simulink model "RegulationSim_v6_N8_5_States"  (R2019b)
settings: Solver=FixedStepAuto  StartTime=0.0  StopTime=100  FixedStep=0.1  RelTol=1e-3
values from neighbouring files (symbols this model uses):
  A = c.A    [MPC_u.m]    (also in base_lab4.m; mpc_regulation.m)
  B = c.B    [MPC_u.m]    (also in base_lab4.m; mpc_regulation.m)
  C = c.C    [MPC_u.m]    (also in base_lab4.m; mpc_regulation.m)
  D = 0    [MPC_u.m]    (also in base_lab4.m; mpc_regulation.m)
undefined symbols (not defined in the file or in its folder): A_new, B_new1, C_new1, D_new1, K1, K2, K3, K4
settings Model: Creator=BHARATHRAJ  LastModifiedBy=Mohan
settings SolverCC: AlgebraicLoopSolver=LineSearch
settings SFSimCC: CustomCodeUndefinedFunction=UseInterfaceOnly

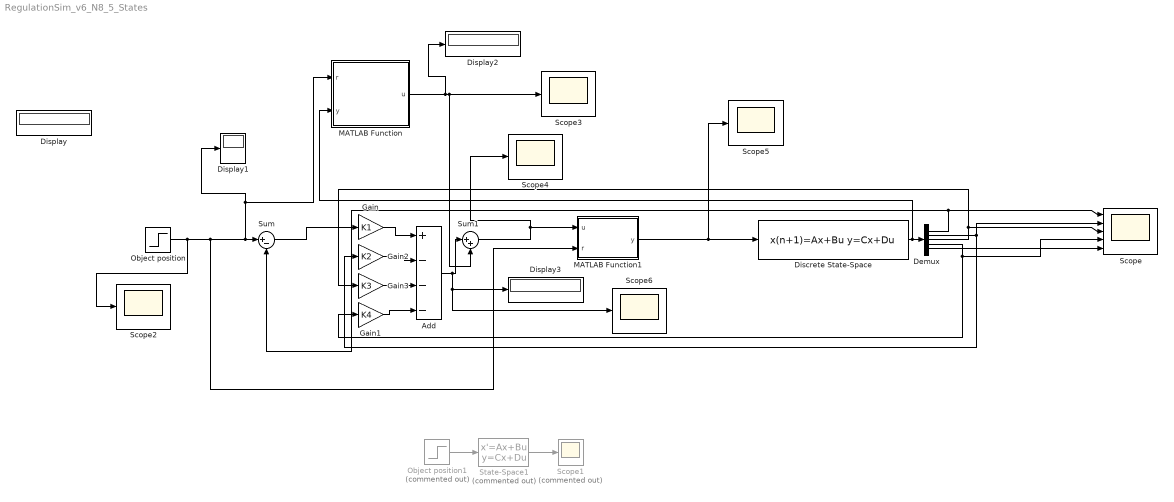
== system RegulationSim_v6_N8_5_States ==
  Add : Sum  Inputs=+---
  Demux : Demux  Outputs=5
  Discrete State-Space : DiscreteStateSpace  A=A_new  B=B_new1  C=C_new1  D=D_new1  InitialCondition=[0 0 0.001 0 0]  SampleTime=-1
  Display{,1..3} (4 alike) : Display
  Gain : Gain  Gain=K1
  Gain1 : Gain  Gain=K4
  Gain2 : Gain  Gain=K2
  Gain3 : Gain  Gain=K3
  MATLAB Function : MATLAB Function  TreatAsAtomicUnit=on
  MATLAB Function1 : MATLAB Function  TreatAsAtomicUnit=on
  Object position : Step  Before=1  SampleTime=0
  Object position1 : Step  Commented=on  SampleTime=0
  Scope : Scope  NumInputPorts=5
  Scope1 : Scope  Commented=on
  Scope{2..6} (5 alike) : Scope
  State-Space1 : StateSpace  Commented=on  A=A  B=B  C=C  D=D  InitialCondition=0
  Sum : Sum  Inputs=|+-
  Sum1 : Sum  Inputs=|++
  wires:
  State-Space1/1 -> Scope1/1
  Object position1/1 -> State-Space1/1
  Demux/1 -> Sum/2, Scope/1
  Demux/2 -> Gain2/1, Scope/2
  Demux/3 -> Scope/3, Gain3/1
  Demux/4 -> Gain1/1, Scope/4
  Discrete State-Space/1 -> MATLAB Function/2(y), Demux/1
  Sum/1 -> Gain/1
  Gain/1 -> Add/1
  Add/1 -> Scope6/1, Display3/1, Sum1/1
  Gain2/1 -> Add/2
  Gain3/1 -> Add/3
  MATLAB Function/1(u) -> Display2/1, Scope3/1, Sum1/2
  Sum1/1 -> MATLAB Function1/1(u), Scope4/1
  Gain1/1 -> Add/4
  Demux/5 -> Scope/5
  MATLAB Function1/1(y) -> Discrete State-Space/1, Scope5/1
  Object position/1 -> Scope2/1, MATLAB Function1/2(r), MATLAB Function/1(r), Display1/1, Sum/1

== matlab function RegulationSim_v6_N8_5_States/MATLAB Function1 ==
  data: u input; y output; r input
function y = fcn(u,r)

y = [u;r;0;0;0];

== matlab function RegulationSim_v6_N8_5_States/MATLAB Function ==
  data: r input; u output; y input
function u = fcn(r,y)
% eml.extrinsic('global')
% global r2
% r2=0;
% r2=r;
m_c=0.493;
m_p=0.312;
I_p=0.00024;
l=0.04;
f1=0.01;
kt=0.11;
R11=10;
r1=0.0335;
g=9.81;
den=I_p*(m_c+m_p)+m_c*m_p*l^2;
A1=[0 1 0 0;0 -(I_p+m_p*l^2)*f1/den m_p^2*g*l^2/den 0;0 0 0 1;0 -m_p*l*f1/den m_p*g*l*(m_c+m_p)/den 0];
B1=[0;(I_p+m_p*l^2)/den;0;m_p*l/den]*(2*kt/(R11*r1));
C1=[1 0 0 0];
D3=0;
Q1=[1e4 0 0 0;0 1 0 0;0 0 8e5 0;0 0 0 1];
R1=1;
N1=0;
eml.extrinsic('lqr')
[K,S1,e] = lqr(A1,B1,Q1,R1,N1);
aa=zeros(4,4);
aa=B1*K;
eml.extrinsic('ss');
a=ss(A1-aa,B1,C1,D3);
eml.extrinsic('c2d')
b=c2d(a,0.005,'zoh');
eml.extrinsic('ssdata')
A=zeros(4,4);
B=zeros(4,1);
C=zeros(1,4);
D=zeros(1,1);
[A,B,C,D] = ssdata(b)

state_n = size(A, 1);
A_new = [A zeros(state_n,1); C 1];
B_new = [B; 0];
C_new = [C 0; zeros(1,state_n) 1];
bb=zeros(4,4)
bb=B*K;
W_new = [bb;-1 0 0 0];
input_n = size(B_new, 2);

N = 8;  %This is the horizon for MPC
R = 0.1;
%RD = 0.1;  %Weight the slew rate - respect actuation bandwidths
Q = diag([5e4; 0]); %Single output
eml.extrinsic('blkdiag')

Qbar = zeros(16,16);
Rbar = zeros(8,8);
eml.extrinsic('blkdiag')
Qbar = blkdiag(Q,Q,Q,Q,Q,Q,Q,Q);
Rbar = blkdiag(R,R,R,R,R,R,R,R);

Tbar = [C_new*A_new ;
        C_new*A_new*A_new ;
        C_new*(A_new^2)*A_new ;
        C_new*(A_new^3)*A_new ;
        C_new*(A_new^4)*A_new ;
        C_new*(A_new^5)*A_new ;
        C_new*(A_new^6)*A_new ;
        C_new*(A_new^7)*A_new ];

Sbar = [C_new*B_new zeros(2,1) zeros(2,1) zeros(2,1) zeros(2,1) zeros(2,1) zeros(2,1) zeros(2,1);
        C_new*A_new*B_new C_new*B_new zeros(2,1) zeros(2,1) zeros(2,1) zeros(2,1) zeros(2,1) zeros(2,1);
        C_new*(A_new^2)*B_new  C_new*A_new*B_new  C_new*B_new zeros(2,1) zeros(2,1) zeros(2,1) zeros(2,1) zeros(2,1);
        C_new*(A_new^3)*B_new C_new*(A_new^2)*B_new C_new*A_new*B_new C_new*B_new zeros(2,1) zeros(2,1) zeros(2,1) zeros(2,1);
        C_new*(A_new^4)*B_new C_new*(A_new^3)*B_new C_new*(A_new^2)*B_new C_new*A_new*B_new C_new*B_new zeros(2,1) zeros(2,1) zeros(2,1);
        C_new*(A_new^5)*B_new C_new*(A_new^4)*B_new C_new*(A_new^3)*B_new C_new*(A_new^2)*B_new C_new*A_new*B_new C_new*B_new zeros(2,1) zeros(2,1);
        C_new*(A_new^6)*B_new C_new*(A_new^5)*B_new C_new*(A_new^4)*B_new C_new*(A_new^3)*B_new C_new*(A_new^2)*B_new C_new*A_new*B_new C_new*B_new zeros(2,1);
        C_new*(A_new^7)*B_new C_new*(A_new^6)*B_new C_new*(A_new^5)*B_new C_new*(A_new^4)*B_new C_new*(A_new^3)*B_new C_new*(A_new^2)*B_new C_new*A_new*B_new C_new*B_new];

Wbar = [C_new*W_new;
        C_new*W_new + C_new*A_new*W_new;
        C_new*W_new + C_new*A_new*W_new + C_new*(A_new^2)*W_new;
        C_new*W_new + C_new*A_new*W_new + C_new*(A_new^2)*W_new + C_new*(A_new^3)*W_new;
        C_new*W_new + C_new*A_new*W_new + C_new*(A_new^2)*W_new + C_new*(A_new^3)*W_new + C_new*(A_new^4)*W_new;
        C_new*W_new + C_new*A_new*W_new + C_new*(A_new^2)*W_new + C_new*(A_new^3)*W_new + C_new*(A_new^4)*W_new + C_new*(A_new^5)*W_new;
        C_new*W_new + C_new*A_new*W_new + C_new*(A_new^2)*W_new + C_new*(A_new^3)*W_new + C_new*(A_new^4)*W_new + C_new*(A_new^5)*W_new + C_new*(A_new^6)*W_new;
        C_new*W_new + C_new*A_new*W_new + C_new*(A_new^2)*W_new + C_new*(A_new^3)*W_new + C_new*(A_new^4)*W_new + C_new*(A_new^5)*W_new + C_new*(A_new^6)*W_new + C_new*(A_new^7)*W_new];
H = (Rbar+Sbar'*Qbar*Sbar);
H = (H+H')/2;

eml.extrinsic('tril')
cc=zeros(N);
cc=tril(eye(N*input_n));
pp=0;
pp=cc
G = [pp;-pp];
S = zeros(2*N*input_n,5);
W = 12*ones(2*N,1);
%RbarD = zeros(10,10);
%Sx = [];
%CAB = [];
% eml.extrinsic('blkdiag')
% eml.extrinsic('sum')
% SU=[];
% Su=zeros(10,10);
% Qbara=zeros(10,10);
% Rbara=zeros(10,10);
% %RbarDa=zeros(10,10);
% r
% for ii = 1:N
%     Qbar(ii,ii) = Q;
%     Rbar(ii,ii) = R;
%     RbarD(ii,ii) = RD;
%     Sx = [Sx;C*A^ii];
%     CAB = [CAB C*A^(ii-1)*B];
% end
% r
% Qbara=Qbar;
% Rbara=Rbar;
% RbarDa=RbarD;
%CAB
% for ii = 1:N
%     %SUU=[];
%     for jj = 1:ii
%         %SUU=[SUU sum(CAB(:,1:ii-jj+1),2)];
%         Su(ii,jj)=sum(CAB(1:ii-jj+1));
%     end
%     %SU = [SUU zeros(4,N-ii)];
%     %Su=[Su;SU];
% end
% Su;
% Su1=zeros(10,1);
% Su1=  Su(:,1);
% eml.extrinsic('tril')
% LL = tril(ones(N));
% LLa=zeros(N,N);
% LLa=LL;
% H = 2*(LLa'*Rbara*LLa+RbarDa+Su'*Qbara*Su);
% eml.extrinsic('diag')
% LR=zeros(10,1);
% LR=diag(LLa'*Rbara')
% Fu = 2*(LR'+Su1'*Qbara*Su)';  %Note the trick on Rbar - u(-1) is really a scalar
% Fr = -2*(Qbara*Su)';
% Fx = 2*(Sx'*Qbara*Su)';
% N1=zeros(N);
% N1=tril(ones(N));
% G = [N1;-N1];
% W0 =12*ones(2*N,1);
% S = zeros(2*N,4);

%X = [0;0;0;0];
X = [0;0;0;0;0];
% v=v+y(1)-r(1);

X=y;
%T =50;
U = 0;
U_disturb = 0;
eml.extrinsic('quadprog')
Z = zeros(N,1);
% options = optimoptions('quadprog');
% options.Display = 'none';
Xact=[];
Uopt=[];
%x0=zeros(100,1)
% for ii = 1:T-1
%     X(1)=y;
%     Xact=[Xact X];
% %     Xact(ii,:) = X;%For graphing
%     r2=r*ones(1,10);
%     f = Fx*X+Fu*U+Fr*(r2-5*ones(1,10))';  %Sometimes people hold r(ii) here
%     W = W0+[ones(N,1)*-U;ones(N,1)*U];
%     Z = quadprog(H,f,G,W+S*X,[],[],[],[],[]);  %Here is the magic!
%     %fun=@(Z)0.5*Z'*H*Z+f'*Z;
%     %Z = fmincon(fun,x0,G,W)
%     Uopt(ii) = U + Z(1);  %Just use the first item  
%     U = Uopt(ii);
%     u=U;
% end
% u =U ;
Rbarref = [r;0;r;0;r;0;r;0;r;0;r;0;r;0;r;0];
RR = [r 0 0 0];
f = 2*(X'*Tbar'*Qbar*Sbar - Rbarref'*Qbar*Sbar - RR*Wbar'*Qbar*Sbar); 
Z = quadprog(H,f,G,W+S*X,[],[],[],[],[]);
Z
u= -Z(1) - U_disturb;


%X = A_new*X + B_new*U + W_new*RR';
% X(1)=y;
% Xact=[Xact X];
% %     Xact(ii,:) = X;%For graphing
% r2=r*ones(1,10);
% r2
% f = Fx*X+Fu*U+Fr*(r2-5*ones(1,10))';  %Sometimes people hold r(ii) here
% f
% W = W0+[ones(N,1)*-U;ones(N,1)*U];
% W
% Z = quadprog(H,f,G,W+S*X,[],[],[],[],[]);  %Here is the magic!
% Z
% %fun=@(Z)0.5*Z'*H*Z+f'*Z;
% %Z = fmincon(fun,x0,G,W)
% U = U + Z(1);  %Just use the first item  
% u=U;
